simulink model "W1P9"  (R2020b)
settings: Solver=VariableStepAuto  StartTime=0.0  StopTime=10.0  RelTol=1e-3
libraries: simulink x6, powerlib x5
settings Model: Creator=saadh  LastModifiedBy=saadh

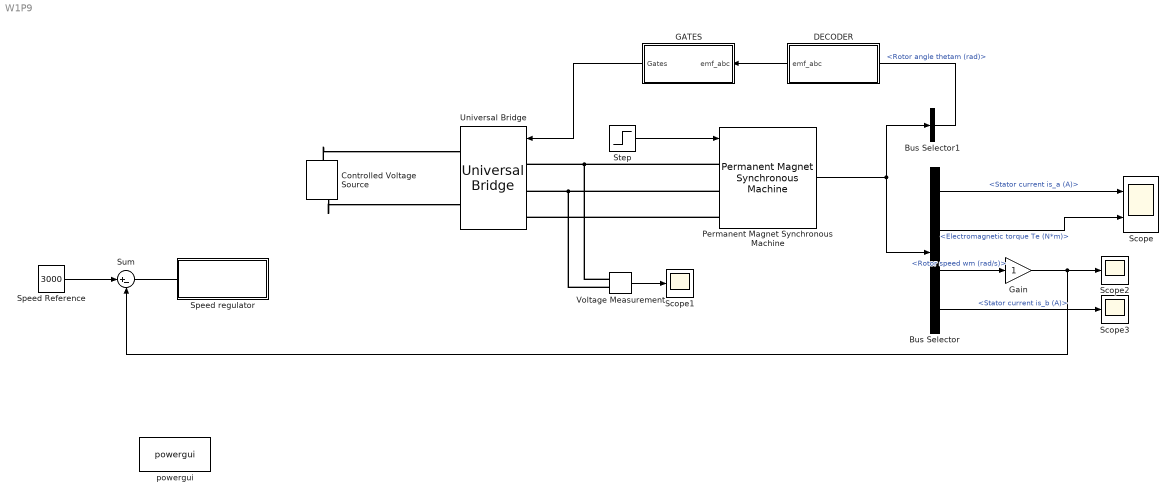
== system W1P9 ==
  Bus Selector : BusSelector  OutputSignals=Stator current is_a (A),Electromagnetic torque Te (N*m),Rotor speed wm (rad/s),Stator current is_b (A)
  Bus Selector1 : BusSelector  OutputSignals=Rotor angle thetam (rad)
  Controlled Voltage Source : powerlib/Electrical Sources/Controlled Voltage Source  Initialize=on  Source_Type=AC  Amplitude=0  Phase=0  Frequency=0  Measurements=None
  DECODER : Subsystem
  GATES : Subsystem
  Gain : Gain
  Permanent Magnet Synchronous Machine : powerlib/Machines/Permanent Magnet Synchronous Machine  NbPhases=3  FluxDistribution=Trapezoidal  RotorType=Round  MechanicalLoad=Torque Tm  PresetModel=No  ShowDetailedParameters=on  MeasurementBus=off  Resistance=0.0485  Inductance=8.5e-3  dqInductances=[8.5e-3,8.5e-3]  La=0.000395  MachineConstant=Flux linkage established by magnets (V.s)  Flux=0.1194  VoltageCst=100.0283  TorqueCst=0.9552  Flat=120  Mechanical=[0.0027 0.0004924 4 0]  PolePairs=4  InitialConditions=[0,0, 0,0]  InitialConditions5ph=[0 0 0 0 0 0]  RefAngle=90 degrees behind phase A axis (modified Park)  IterativeDiscreteModel=Trapezoidal non iterative  TsBlock=-1  TsPowergui=0
  Scope : Scope  NumInputPorts=2
  Scope1 : Scope
  Scope2 : Scope
  Scope3 : Scope
  Speed Reference : Constant  Value=3000
  Speed regulator : Subsystem
  Step : Step  SampleTime=0
  Sum : Sum  Inputs=|+-
  Universal Bridge : powerlib/Power Electronics/Universal Bridge  Arms=3  SnubberResistance=1e5  SnubberCapacitance=inf  Device=MOSFET / Diodes  Ron=1e-3  Lon=0  ForwardVoltages="[  0  0  ]"  ForwardVoltage=0  GTOparameters=[ 10e-6 , 20e-6 ]  IGBTparameters=[ 1e-6 , 2e-6 ]  Measurements=None  Measurements_2=None  converterType=Rectifier
  Voltage Measurement : powerlib/Measurements/Voltage Measurement  PhasorSimulation=off  OutputType=Complex  PSBequivalent=0
  powergui : powerlib/powergui  Priority=1  SimulationMode=Discrete  SampleTime=50e-6  frequency=60  Iterations=50  frequencyindice=60  Pbase=100e6  ErrMax=1e-4  UnitsV=kV  UnitsW=MW  buscounter=0  FunctionMessages=off  echomessages=off  EnableUseOfTLC=off  CurrentSourceSwitches=off  DisableSnubberDevices=off  DisableRonSwitches=off  DisableVfSwitches=off  DisplayEquations=off  AutomaticDiscreteSolvers=off  SolverType=Tustin/Backward Euler (TBE)  Interpol=off  ExternalGateDelay=off  methode=off  Ts=100  x0status=blocks  SPID=on  SwTol=0  HookPort=off  NonlinearTolerance=1e-4  nMaxIteration=100  ContinueOnMaxIteration=off  RestoreLinks=warning  ResistiveCurrentMeasurement=off  Frange=[0:2:500]  Ylog=off  Xlog=on  ShowGrid=off  save=off  variable=ZData  structure=0  ZoomFFT=off  StartTime=0.0  cycles=1  DisplayStyle=1  fundamental=60  FreqAxis=off  MaxFrequency=1000  frequencyindicesteady=1  RmsSteady=1  display=off
  wires:
  ? -> Controlled Voltage Source/1
  Sum/1 -> ?
  Speed Reference/1 -> Sum/1
  DECODER/1(emf_abc) -> GATES/1(emf_abc)
  GATES/1(Gates) -> Universal Bridge/1
  Step/1 -> Permanent Magnet Synchronous Machine/1
  Permanent Magnet Synchronous Machine/1 -> Bus Selector1/1, Bus Selector/1
  Bus Selector1/1 -> ?  "<Rotor angle thetam (rad)>"
  Bus Selector/1 -> Scope/1  "<Stator current is_a (A)>"
  Bus Selector/2 -> Scope/2  "<Electromagnetic torque Te (N*m)>"
  Bus Selector/3 -> Gain/1  "<Rotor speed wm (rad/s)>"
  Bus Selector/4 -> Scope3/1  "<Stator current is_b (A)>"
  Gain/1 -> Sum/2, Scope2/1
  Voltage Measurement/1 -> Scope1/1
  connections:
  Permanent Magnet Synchronous Machine/LConn2 -- Voltage Measurement/LConn2 -- Universal Bridge/LConn2
  Permanent Magnet Synchronous Machine/LConn1 -- Voltage Measurement/LConn1 -- Universal Bridge/LConn1
  Permanent Magnet Synchronous Machine/LConn3 -- Universal Bridge/LConn3
  Controlled Voltage Source/RConn1 -- Universal Bridge/RConn1
  Controlled Voltage Source/LConn1 -- Universal Bridge/RConn2

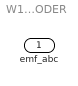
== system W1P9/DECODER ==
  emf_abc : Outport

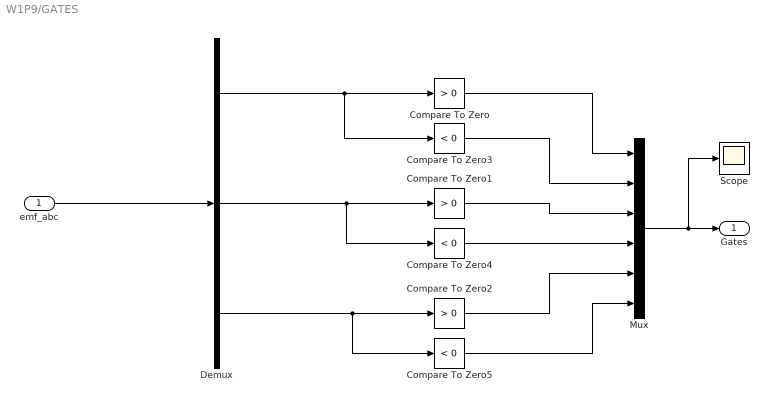
== system W1P9/GATES ==
  emf_abc : Inport
  Compare To Zero : simulink/Logic and Bit Operations/Compare To Zero  relop=>  OutDataTypeStr=boolean
  Compare To Zero1 : simulink/Logic and Bit Operations/Compare To Zero  relop=>  OutDataTypeStr=boolean
  Compare To Zero2 : simulink/Logic and Bit Operations/Compare To Zero  relop=>  OutDataTypeStr=boolean
  Compare To Zero3 : simulink/Logic and Bit Operations/Compare To Zero  relop=<  OutDataTypeStr=boolean
  Compare To Zero4 : simulink/Logic and Bit Operations/Compare To Zero  relop=<  OutDataTypeStr=boolean
  Compare To Zero5 : simulink/Logic and Bit Operations/Compare To Zero  relop=<  OutDataTypeStr=boolean
  Demux : Demux  Outputs=3
  Mux : Mux  Inputs=6
  Scope : Scope
  Gates : Outport
  wires:
  Demux/1 -> Compare To Zero3/1, Compare To Zero/1
  Demux/2 -> Compare To Zero4/1, Compare To Zero1/1
  Demux/3 -> Compare To Zero5/1, Compare To Zero2/1
  Compare To Zero4/1 -> Mux/4
  Compare To Zero1/1 -> Mux/3
  Compare To Zero3/1 -> Mux/2
  Compare To Zero/1 -> Mux/1
  Compare To Zero2/1 -> Mux/5
  Compare To Zero5/1 -> Mux/6
  Mux/1 -> Scope/1, Gates/1
  emf_abc/1 -> Demux/1

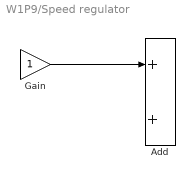
== system W1P9/Speed regulator ==
  Add : Sum
  Gain : Gain
  wires:
  Gain/1 -> Add/1
